simulink model "Perturbatiedebitintrare"  (R2024b)
settings: Solver=VariableStepAuto  StartTime=0.0  StopTime=1000  RelTol=1e-3
values from neighbouring files (symbols this model uses):
  A = 332.5    [scriptProiect.m]
  C = 9    [scriptProiect.m]
  h0 = 10.5    [scriptProiect.m]
  k = 0.035    [scriptProiect.m]
  k1 = 0.624    [scriptProiect.m]
  k11 = k2^2 + 4*(k-k3)*k1    (= 0.0890826)    [scriptProiect.m]
  k12 = 8 * (k-k3)    (= 0.2848)    [scriptProiect.m]
  k13 = 2 * (k-k3)    (= 0.0712)    [scriptProiect.m]
  k2 = -0.015    [scriptProiect.m]
  k3 = -0.0006    [scriptProiect.m]
  keta = 8 * 10^-5    (= 8e-05)    [scriptProiect.m]
  KR = Tp/T0/kp    (= 2.40963855422)    [scriptProiect.m]
  q0 = 29.2    [scriptProiect.m]
  Rm = 3    [scriptProiect.m]
  Ti = Tp    (= 154)    [scriptProiect.m]
libraries: slpidlib x2
settings Model: Creator=Teo  LastModifiedBy=Teo

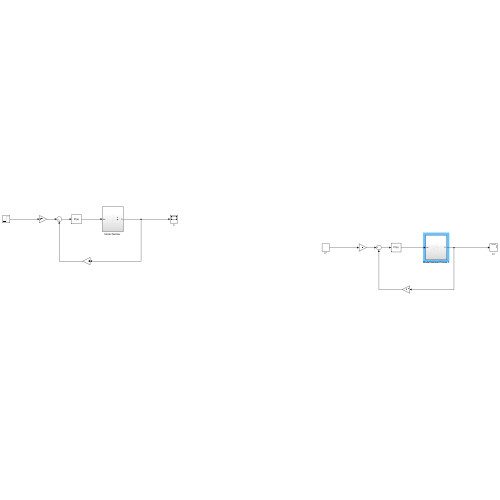
[thumbnail: Simulink's stored preview of the top-level diagram]
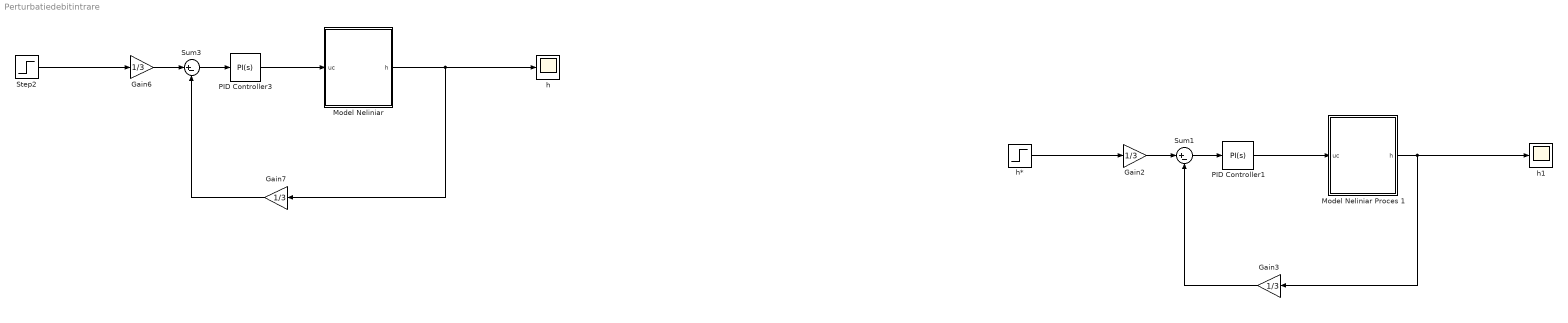
== system Perturbatiedebitintrare ==
  Gain{2..3,6..7} (4 alike) : Gain  Gain=1/3
  "Model Neliniar " : Subsystem
  Model Neliniar Proces 1 : Subsystem
  PID Controller1 : slpidlib/PID Controller  Controller=PI  Form=Parallel  TimeDomain=Continuous-time  UseExternalTs=off  SampleTime=-1  IntegratorMethod=Forward Euler  FilterMethod=Forward Euler  ControllerParametersSource=internal  P=KR  I=KR/Ti  UseKiTs=off  D=0  UseExternalDerivativeSource=off  N=100  UseFilter=on  TunerSelectOption=Transfer Function Based (PID Tuner App)  InitialConditionSource=internal  InitialConditionForIntegrator=5  InitialConditionForFilter=0  DifferentiatorICPrevScaledInput=0  ExternalReset=none  TrackingMode=off  Kt=1  LimitOutput=off  SatLimitsSource=internal  UpperSaturationLimit=inf  LowerSaturationLimit=-inf  LinearizeAsGain=on  AntiWindupMode=none  Kb=1  LimitIntegrator=off  UpperIntegratorSaturationLimit=inf  LowerIntegratorSaturationLimit=-inf  POutMin=[]  POutMax=[]  IOutMin=[]  IOutMax=[]  DOutMin=[]  DOutMax=[]  NOutMin=[]  NOutMax=[]  SumOutMin=[]  SumOutMax=[]  SaturationOutMin=[]  SaturationOutMax=[]  PParamMin=[]  PParamMax=[]  IParamMin=[]  IParamMax=[]  DParamMin=[]  DParamMax=[]  NParamMin=[]  NParamMax=[]  KbParamMin=[]  KbParamMax=[]  KtParamMin=[]  KtParamMax=[]  KbOutMin=[]  KbOutMax=[]  KtOutMin=[]  KtOutMax=[]  IntegratorOutMin=[]  IntegratorOutMax=[]  FilterOutMin=[]  FilterOutMax=[]  SumI1OutMin=[]  SumI1OutMax=[]  SumI2OutMin=[]  SumI2OutMax=[]  SumI3OutMin=[]  SumI3OutMax=[]  SumI4OutMin=[]  SumI4OutMax=[]  SumDOutMin=[]  SumDOutMax=[]  DifferentiatorOutMin=[]  DifferentiatorOutMax=[]  FilterDiffOutCoefMin=[]  FilterDiffOutCoefMax=[]  ReciprocalOutMin=[]  ReciprocalOutMax=[]  SumDenOutMin=[]  SumDenOutMax=[]  SumNumOutMin=[]  SumNumOutMax=[]  DivideOutMin=[]  DivideOutMax=[]  UdiffTsProdOutMin=[]  UdiffTsProdOutMax=[]  NTsProdOutMin=[]  NTsProdOutMax=[]  UintegralTsProdOutMin=[]  UintegralTsProdOutMax=[]  UngainTsProdOutMin=[]  UngainTsProdOutMax=[]  ClampingZeroOutDataTypeStr=Inherit: Inherit via back propagation  ClampingZeroOutMin=[]  ClampingZeroOutMax=[]  FilterDenConstantOutDataTypeStr=Inherit: Inherit via back propagation  FilterDenConstantOutMin=[]  FilterDenConstantOutMax=[]  PCopyOutDataTypeStr=Inherit: Inherit via back propagation  PCopyOutMin=[]  PCopyOutMax=[]  NCopyOutDataTypeStr=Inherit: Inherit via back propagation  NCopyOutMin=[]  NCopyOutMax=[]  IntegratorContinuousStateAttributes=''  IntegratorStateMustResolveToSignalObject=off  IntegratorRTWStateStorageClass=Auto  FilterContinuousStateAttributes=''  FilterStateMustResolveToSignalObject=off  FilterRTWStateStorageClass=Auto  ParallelPVariant=InternalParameters  IdealPVariant=Disabled  IVariant=InternalParameters  DVariant=Disabled  IntegratorVariant=Continuous  SatVariant=Disabled  AWVariant=Passthrough  PCopyVariant=Disabled  TRVariant=Disabled  FdbkBlocksVariant=Forward  IdealPFdbkVariant=Disabled  SatFdbkVariant=Disabled  DerivativeFilterVariant=Disabled  NVariant=Disabled  NCopyVariant=Disabled_SignalSpec  FilterICVariant=Disabled  IntegratorICVariant=InternalICs  ExternalResetVariant=Disabled  TRSumVariant=Passthrough  SumFdbkVariant=Disabled  SumVariant=Sum_PI  TsampFilterVariant=InternalTs  TsampNgainVariant=Passthrough  TsampIntegralVariant=Disabled_SignalSpec  ExternalSaturationOutDataTypeStr=Inherit: Same as second input  DerivativeSourceVariant=Disabled  PreIntVariant=InternalPreInt
  PID Controller3 : slpidlib/PID Controller  Controller=PI  Form=Parallel  TimeDomain=Continuous-time  UseExternalTs=off  SampleTime=-1  IntegratorMethod=Forward Euler  FilterMethod=Forward Euler  ControllerParametersSource=internal  P=KR  I=KR/Ti  UseKiTs=off  D=0  UseExternalDerivativeSource=off  N=100  UseFilter=on  TunerSelectOption=Transfer Function Based (PID Tuner App)  InitialConditionSource=internal  InitialConditionForIntegrator=5  InitialConditionForFilter=0  DifferentiatorICPrevScaledInput=0  ExternalReset=none  TrackingMode=off  Kt=1  LimitOutput=off  SatLimitsSource=internal  UpperSaturationLimit=inf  LowerSaturationLimit=-inf  LinearizeAsGain=on  AntiWindupMode=none  Kb=1  LimitIntegrator=off  UpperIntegratorSaturationLimit=inf  LowerIntegratorSaturationLimit=-inf  POutMin=[]  POutMax=[]  IOutMin=[]  IOutMax=[]  DOutMin=[]  DOutMax=[]  NOutMin=[]  NOutMax=[]  SumOutMin=[]  SumOutMax=[]  SaturationOutMin=[]  SaturationOutMax=[]  PParamMin=[]  PParamMax=[]  IParamMin=[]  IParamMax=[]  DParamMin=[]  DParamMax=[]  NParamMin=[]  NParamMax=[]  KbParamMin=[]  KbParamMax=[]  KtParamMin=[]  KtParamMax=[]  KbOutMin=[]  KbOutMax=[]  KtOutMin=[]  KtOutMax=[]  IntegratorOutMin=[]  IntegratorOutMax=[]  FilterOutMin=[]  FilterOutMax=[]  SumI1OutMin=[]  SumI1OutMax=[]  SumI2OutMin=[]  SumI2OutMax=[]  SumI3OutMin=[]  SumI3OutMax=[]  SumI4OutMin=[]  SumI4OutMax=[]  SumDOutMin=[]  SumDOutMax=[]  DifferentiatorOutMin=[]  DifferentiatorOutMax=[]  FilterDiffOutCoefMin=[]  FilterDiffOutCoefMax=[]  ReciprocalOutMin=[]  ReciprocalOutMax=[]  SumDenOutMin=[]  SumDenOutMax=[]  SumNumOutMin=[]  SumNumOutMax=[]  DivideOutMin=[]  DivideOutMax=[]  UdiffTsProdOutMin=[]  UdiffTsProdOutMax=[]  NTsProdOutMin=[]  NTsProdOutMax=[]  UintegralTsProdOutMin=[]  UintegralTsProdOutMax=[]  UngainTsProdOutMin=[]  UngainTsProdOutMax=[]  ClampingZeroOutDataTypeStr=Inherit: Inherit via back propagation  ClampingZeroOutMin=[]  ClampingZeroOutMax=[]  FilterDenConstantOutDataTypeStr=Inherit: Inherit via back propagation  FilterDenConstantOutMin=[]  FilterDenConstantOutMax=[]  PCopyOutDataTypeStr=Inherit: Inherit via back propagation  PCopyOutMin=[]  PCopyOutMax=[]  NCopyOutDataTypeStr=Inherit: Inherit via back propagation  NCopyOutMin=[]  NCopyOutMax=[]  IntegratorContinuousStateAttributes=''  IntegratorStateMustResolveToSignalObject=off  IntegratorRTWStateStorageClass=Auto  FilterContinuousStateAttributes=''  FilterStateMustResolveToSignalObject=off  FilterRTWStateStorageClass=Auto  ParallelPVariant=InternalParameters  IdealPVariant=Disabled  IVariant=InternalParameters  DVariant=Disabled  IntegratorVariant=Continuous  SatVariant=Disabled  AWVariant=Passthrough  PCopyVariant=Disabled  TRVariant=Disabled  FdbkBlocksVariant=Forward  IdealPFdbkVariant=Disabled  SatFdbkVariant=Disabled  DerivativeFilterVariant=Disabled  NVariant=Disabled  NCopyVariant=Disabled_SignalSpec  FilterICVariant=Disabled  IntegratorICVariant=InternalICs  ExternalResetVariant=Disabled  TRSumVariant=Passthrough  SumFdbkVariant=Disabled  SumVariant=Sum_PI  TsampFilterVariant=InternalTs  TsampNgainVariant=Passthrough  TsampIntegralVariant=Disabled_SignalSpec  ExternalSaturationOutDataTypeStr=Inherit: Same as second input  DerivativeSourceVariant=Disabled  PreIntVariant=InternalPreInt
  Step2 : Step  Time=0  After=13  SampleTime=0
  Sum1 : Sum  Inputs=|+-
  Sum3 : Sum  Inputs=|+-
  h : Scope
  h* : Step  Time=0  After=13  SampleTime=0
  h1 : Scope
  wires:
  Step2/1 -> Gain6/1
  Gain6/1 -> Sum3/1
  Gain7/1 -> Sum3/2
  PID Controller3/1 -> "Model Neliniar "/1(uc)
  Sum3/1 -> PID Controller3/1
  "Model Neliniar "/1(h) -> Gain7/1, h/1
  Model Neliniar Proces 1/1(h) -> Gain3/1, h1/1
  PID Controller1/1 -> Model Neliniar Proces 1/1(uc)
  Gain3/1 -> Sum1/2
  Sum1/1 -> PID Controller1/1
  h*/1 -> Gain2/1
  Gain2/1 -> Sum1/1

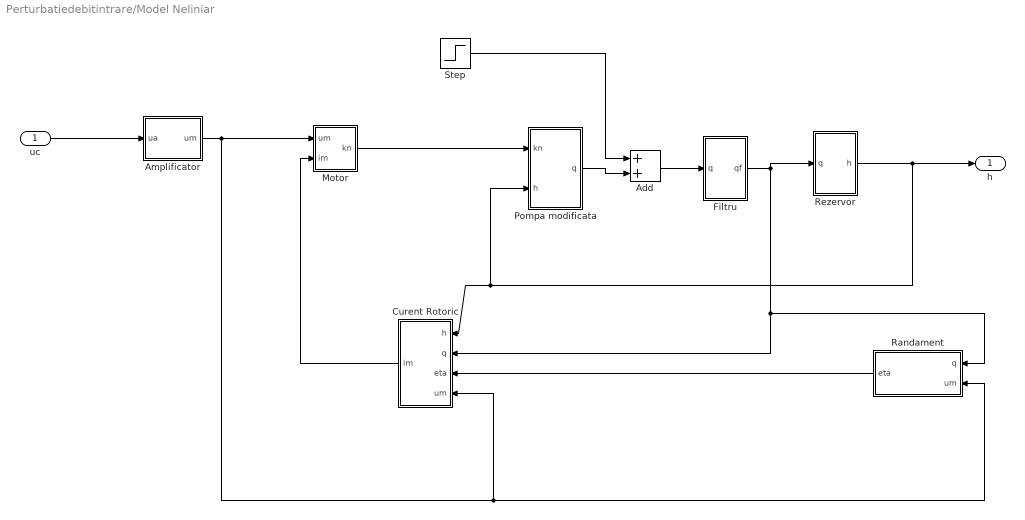
== system Perturbatiedebitintrare/Model Neliniar  ==
  uc : Inport
  Add : Sum
  Amplificator : Subsystem
  Curent Rotoric : Subsystem
  Filtru : Subsystem
  Motor : Subsystem
  Pompa modificata : Subsystem
  "Randament " : Subsystem
  Rezervor : Subsystem
  Step : Step  Time=500  After=0.3* q0  SampleTime=0
  h : Outport
  wires:
  Rezervor/1(h) -> h/1, Pompa modificata/2(h), Curent Rotoric/1(h)
  uc/1 -> Amplificator/1(ua)
  "Randament "/1(eta) -> Curent Rotoric/3(eta)
  Curent Rotoric/1(im) -> Motor/2(im)
  Filtru/1(qf) -> Rezervor/1(q), "Randament "/1(q), Curent Rotoric/2(q)
  Amplificator/1(um) -> Curent Rotoric/4(um), "Randament "/2(um), Motor/1(um)
  Motor/1(kn) -> Pompa modificata/1(kn)
  Add/1 -> Filtru/1(q)
  Pompa modificata/1(q) -> Add/2
  Step/1 -> Add/1

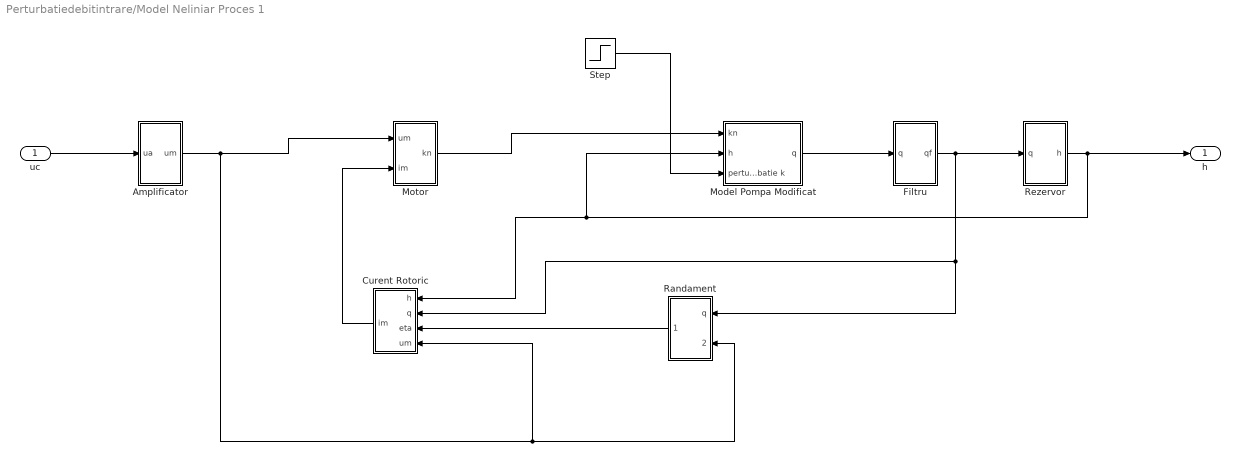
== system Perturbatiedebitintrare/Model Neliniar Proces 1 ==
  uc : Inport
  Amplificator : Subsystem
  Curent Rotoric : Subsystem
  Filtru : Subsystem
  Model Pompa Modificat : Subsystem
  Motor : Subsystem
  "Randament " : Subsystem
  Rezervor : Subsystem
  Step : Step  Time=250  After=0.3*k  SampleTime=0
  h : Outport
  wires:
  Curent Rotoric/1(im) -> Motor/2(im)
  "Randament "/1(eta) -> Curent Rotoric/3(eta)
  Motor/1(kn) -> Model Pompa Modificat/1(kn)
  Rezervor/1(h) -> h/1, Curent Rotoric/1(h), Model Pompa Modificat/2(h)
  Filtru/1(qf) -> "Randament "/1(q), Curent Rotoric/2(q), Rezervor/1(q)
  uc/1 -> Amplificator/1(ua)
  Amplificator/1(um) -> "Randament "/2(um), Curent Rotoric/4(um), Motor/1(um)
  Model Pompa Modificat/1(q) -> Filtru/1(q)
  Step/1 -> Model Pompa Modificat/3(perturbatie k)

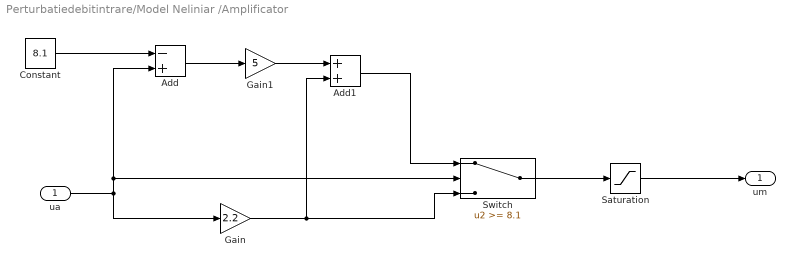
== system Perturbatiedebitintrare/Model Neliniar /Amplificator ==
  ua : Inport
  Add : Sum  Inputs=-+
  Add1 : Sum
  Constant : Constant  Value=8.1
  Gain : Gain  Gain=2.2
  Gain1 : Gain  Gain=5
  Saturation : Saturate  UpperLimit=22  LowerLimit=0
  Switch : Switch  Threshold=8.1  SaturateOnIntegerOverflow=off  InputSameDT=off
  um : Outport
  wires:
  Constant/1 -> Add/1
  ua/1 -> Add/2, Switch/2, Gain/1
  Add/1 -> Gain1/1
  Add1/1 -> Switch/1
  Switch/1 -> Saturation/1
  Gain/1 -> Switch/3, Add1/2
  Gain1/1 -> Add1/1
  Saturation/1 -> um/1

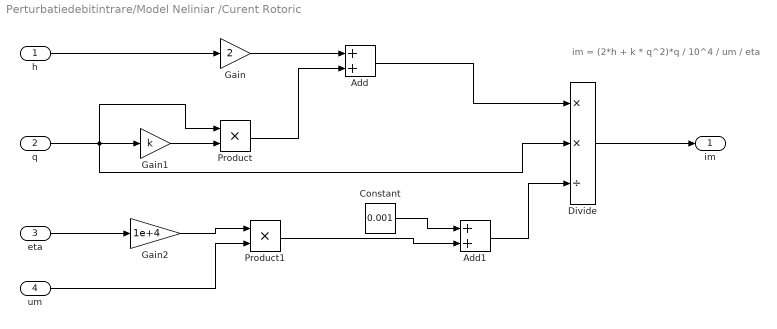
== system Perturbatiedebitintrare/Model Neliniar /Curent Rotoric ==
  note: im = (2*h + k * q^2)*q / 10^4 / um / eta
  h : Inport
  q : Inport  Port=2
  eta : Inport  Port=3
  um : Inport  Port=4
  Add : Sum
  Add1 : Sum
  Constant : Constant  Value=0.001
  Divide : Product  Inputs=**/
  Gain : Gain  Gain=2
  Gain1 : Gain  Gain=k
  Gain2 : Gain  Gain=1e+4
  Product : Product
  Product1 : Product
  im : Outport
  wires:
  Add/1 -> Divide/1
  Constant/1 -> Add1/1
  Add1/1 -> Divide/3
  q/1 -> Divide/2, Product/1, Gain1/1
  Gain/1 -> Add/1
  eta/1 -> Gain2/1
  h/1 -> Gain/1
  Gain1/1 -> Product/2
  Product1/1 -> Add1/2
  Divide/1 -> im/1
  um/1 -> Product1/2
  Product/1 -> Add/2
  Gain2/1 -> Product1/1

== system Perturbatiedebitintrare/Model Neliniar /Filtru ==
  q : Inport
  Integrator : Integrator
  Sum : Sum  Inputs=|+-
  qf : Outport
  wires:
  Integrator/1 -> qf/1, Sum/2
  Sum/1 -> Integrator/1
  q/1 -> Sum/1

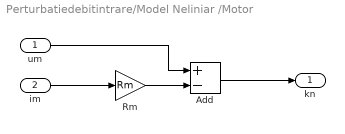
== system Perturbatiedebitintrare/Model Neliniar /Motor ==
  um : Inport
  im : Inport  Port=2
  Add : Sum  Inputs=+-
  Rm : Gain  Gain=Rm
  kn : Outport
  wires:
  um/1 -> Add/1
  Rm/1 -> Add/2
  Add/1 -> kn/1
  im/1 -> Rm/1

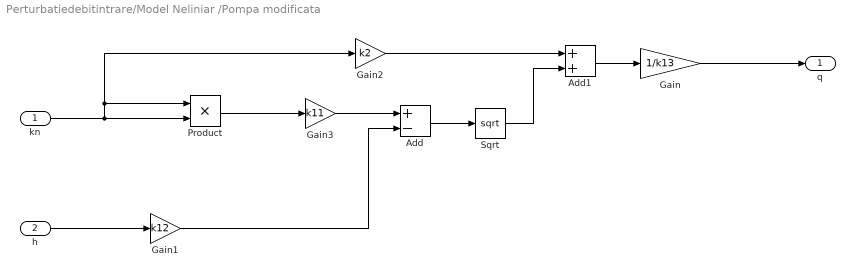
== system Perturbatiedebitintrare/Model Neliniar /Pompa modificata ==
  kn : Inport
  h : Inport  Port=2
  Add : Sum  Inputs=+-
  Add1 : Sum
  Gain : Gain  Gain=1/k13
  Gain1 : Gain  Gain=k12
  Gain2 : Gain  Gain=k2
  Gain3 : Gain  Gain=k11
  Product : Product
  Sqrt : Sqrt
  q : Outport
  wires:
  kn/1 -> Product/1, Gain2/1, Product/2
  Gain3/1 -> Add/1
  Product/1 -> Gain3/1
  Add1/1 -> Gain/1
  h/1 -> Gain1/1
  Gain2/1 -> Add1/1
  Add/1 -> Sqrt/1
  Sqrt/1 -> Add1/2
  Gain1/1 -> Add/2
  Gain/1 -> q/1

== system Perturbatiedebitintrare/Model Neliniar /Randament  ==
  q : Inport
  um : Inport  Port=2
  Gain : Gain  Gain=keta
  Product : Product
  eta : Outport
  wires:
  q/1 -> Product/1
  Product/1 -> eta/1
  Gain/1 -> Product/2
  um/1 -> Gain/1

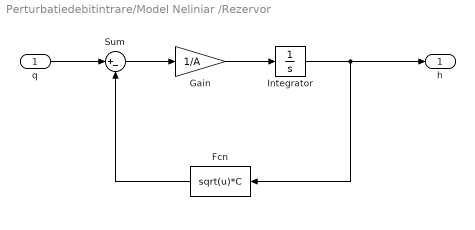
== system Perturbatiedebitintrare/Model Neliniar /Rezervor ==
  q : Inport
  Fcn : Fcn  Expr=sqrt(u)*C
  Gain : Gain  Gain=1/A
  Integrator : Integrator
  Sum : Sum  Inputs=|+-
  h : Outport
  wires:
  Gain/1 -> Integrator/1
  q/1 -> Sum/1
  Sum/1 -> Gain/1
  Integrator/1 -> h/1, Fcn/1
  Fcn/1 -> Sum/2

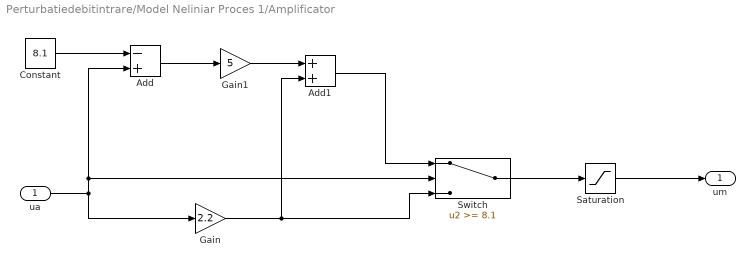
== system Perturbatiedebitintrare/Model Neliniar Proces 1/Amplificator ==
  ua : Inport
  Add : Sum  Inputs=-+
  Add1 : Sum
  Constant : Constant  Value=8.1
  Gain : Gain  Gain=2.2
  Gain1 : Gain  Gain=5
  Saturation : Saturate  UpperLimit=22  LowerLimit=0
  Switch : Switch  Threshold=8.1  SaturateOnIntegerOverflow=off  InputSameDT=off
  um : Outport
  wires:
  Add/1 -> Gain1/1
  Add1/1 -> Switch/1
  Switch/1 -> Saturation/1
  Constant/1 -> Add/1
  Saturation/1 -> um/1
  Gain/1 -> Switch/3, Add1/2
  ua/1 -> Add/2, Switch/2, Gain/1
  Gain1/1 -> Add1/1

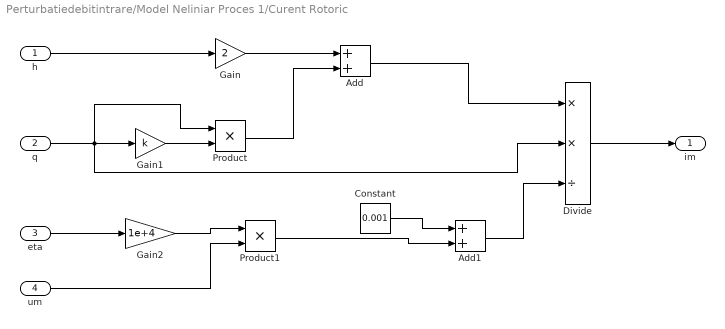
== system Perturbatiedebitintrare/Model Neliniar Proces 1/Curent Rotoric ==
  h : Inport
  q : Inport  Port=2
  eta : Inport  Port=3
  um : Inport  Port=4
  Add : Sum
  Add1 : Sum
  Constant : Constant  Value=0.001
  Divide : Product  Inputs=**/
  Gain : Gain  Gain=2
  Gain1 : Gain  Gain=k
  Gain2 : Gain  Gain=1e+4
  Product : Product
  Product1 : Product
  im : Outport
  wires:
  Gain1/1 -> Product/2
  Gain/1 -> Add/1
  Gain2/1 -> Product1/1
  q/1 -> Divide/2, Product/1, Gain1/1
  Add1/1 -> Divide/3
  Product1/1 -> Add1/2
  um/1 -> Product1/2
  Add/1 -> Divide/1
  Product/1 -> Add/2
  eta/1 -> Gain2/1
  h/1 -> Gain/1
  Constant/1 -> Add1/1
  Divide/1 -> im/1

== system Perturbatiedebitintrare/Model Neliniar Proces 1/Filtru ==
  q : Inport
  Integrator : Integrator  InitialCondition=q0
  Sum : Sum  Inputs=|+-
  qf : Outport
  wires:
  q/1 -> Sum/1
  Integrator/1 -> qf/1, Sum/2
  Sum/1 -> Integrator/1

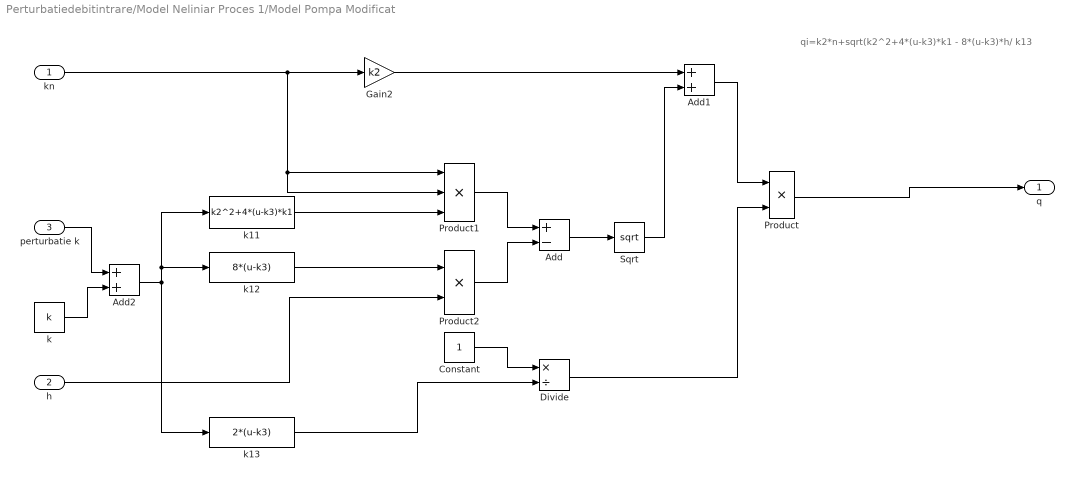
== system Perturbatiedebitintrare/Model Neliniar Proces 1/Model Pompa Modificat ==
  note: qi=k2*n+sqrt(k2^2+4*(u-k3)*k1 - 8*(u-k3)*h/ k13
  kn : Inport
  h : Inport  Port=2
  perturbatie k : Inport  Port=3
  Add : Sum  Inputs=+-
  Add1 : Sum
  Add2 : Sum
  Constant : Constant
  Divide : Product  Inputs=*/
  Gain2 : Gain  Gain=k2
  Product : Product
  Product1 : Product  Inputs=3
  Product2 : Product
  Sqrt : Sqrt
  k : Constant  Value=k
  k11 : Fcn  Expr=k2^2+4*(u-k3)*k1
  k12 : Fcn  Expr=8*(u-k3)
  k13 : Fcn  Expr=2*(u-k3)
  q : Outport
  wires:
  h/1 -> Product2/2
  Sqrt/1 -> Add1/2
  Add1/1 -> Product/1
  Add/1 -> Sqrt/1
  Gain2/1 -> Add1/1
  kn/1 -> Product1/2, Product1/1, Gain2/1
  Product1/1 -> Add/1
  Product2/1 -> Add/2
  perturbatie k/1 -> Add2/1
  k/1 -> Add2/2
  Add2/1 -> k12/1, k11/1, k13/1
  k11/1 -> Product1/3
  k12/1 -> Product2/1
  Constant/1 -> Divide/1
  k13/1 -> Divide/2
  Divide/1 -> Product/2
  Product/1 -> q/1

== system Perturbatiedebitintrare/Model Neliniar Proces 1/Motor ==
  note: Rm=rezistența înfașurării rotorice a motorului
  um : Inport
  im : Inport  Port=2
  Add : Sum  Inputs=+-
  Rm : Gain  Gain=Rm
  kn : Outport
  wires:
  im/1 -> Rm/1
  Rm/1 -> Add/2
  um/1 -> Add/1
  Add/1 -> kn/1

== system Perturbatiedebitintrare/Model Neliniar Proces 1/Randament  ==
  note: eta=𝑘eta*𝑢𝑚*𝑞
      | um=tensiune alimentare
      | q=debit pompa
      | keta = 8∗10−5
  q : Inport
  um : Inport  Port=2
  Gain : Gain  Gain=keta
  Product : Product
  eta : Outport
  wires:
  um/1 -> Gain/1
  Product/1 -> eta/1
  Gain/1 -> Product/2
  q/1 -> Product/1

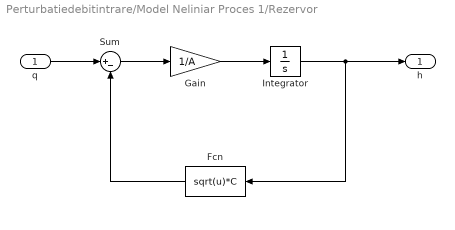
== system Perturbatiedebitintrare/Model Neliniar Proces 1/Rezervor ==
  q : Inport
  Fcn : Fcn  Expr=sqrt(u)*C
  Gain : Gain  Gain=1/A
  Integrator : Integrator  InitialCondition=h0
  Sum : Sum  Inputs=|+-
  h : Outport
  wires:
  Fcn/1 -> Sum/2
  Gain/1 -> Integrator/1
  Sum/1 -> Gain/1
  Integrator/1 -> h/1, Fcn/1
  q/1 -> Sum/1
